simulink model "HybridEngModel"  (R2013a)
settings: Solver=ode15s  StartTime=0  StopTime=100  FixedStep=1e-3  RelTol=1e-5  AbsTol=1e-5
values from neighbouring files (symbols this model uses):
  B = [B1;B2]    [GensetRespOptimiztion.m]    (also in GensetRespOptimiztionTorstein.m; Init8RTFLEX68D.m = 0.68; init_MVM.m = 0.127)
  beta = 0.75    [Init8RTFLEX68D.m]
  cAStartRef = 104.8    [Init8RTFLEX68D.m]
  dCALiftDown = cAVVDownRef(end) - cAVVDownRef(1)    [Init8RTFLEX68D.m]
  dCALiftTopRef = 63.5    [Init8RTFLEX68D.m]
  dCALiftUp = cAVVUpRef(end) - cAVVUpRef(1)    [Init8RTFLEX68D.m]
  Dp = 0.383    [Init8RTFLEX68D.m]
  Ds = 0.079    [Init8RTFLEX68D.m]
  Dv = 0.425    [Init8RTFLEX68D.m]
  liftMax = 0.17    [Init8RTFLEX68D.m]
  nStroke = 2    [Init8RTFLEX68D.m]
  w = 0.021    [Init8RTFLEX68D.m]
  wNL0 = 1./(1-Droop*.5)    [initHybrid.m]    (also in initMV.m; init_ele.m = 1.0101010101)
undefined symbols (not defined in the file or in its folder): cAVVDownRef, cAVVUpRef, generators, liftDownRef, liftUpRef
undefined symbols (not defined in the file): aCrank, cAlpha, cCylHT, E0A, ECyl0, fs, hn, lambdaCrank, m0A, mb0A, mbCyl0, mCp, mCyl0, mqfCycMax, nCyl, nPort, phi0, phi0A, r, stroke, V0A, vCyl0, wiebePara, X, Y
libraries: EngineSystemSubmodel x15, simulink x1, gensetMV x1
settings Model: Creator=yum  LastModifiedBy=yum
settings DataIOCC: SaveFormat=StructureWithTime  InspectSignalLogs=on  ReturnWorkspaceOutputs=on
settings DebuggingCC: SolverPrmCheckMsg=none

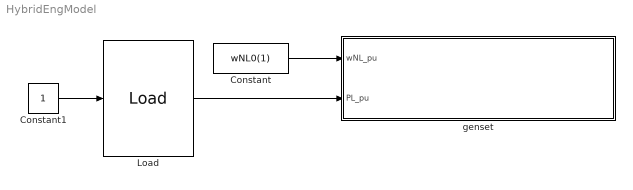
== system HybridEngModel ==
  Constant : Constant  Value=wNL0(1)
  Constant1 : Constant
  Load : EngineSystemSubmodel/Load  Load_index=Load_index  Load_amp=Load_amp  Load_bias=Load_bias  Start_time=Start_time  T_load=T_load
  genset : Subsystem  mask{genset=generators(1)}
      mask prompts: genset "Generator parameters"
  wires:
  Load/1 -> genset/2(PL_pu)
  Constant/1 -> genset/1(wNL_pu)
  Constant1/1 -> Load/1

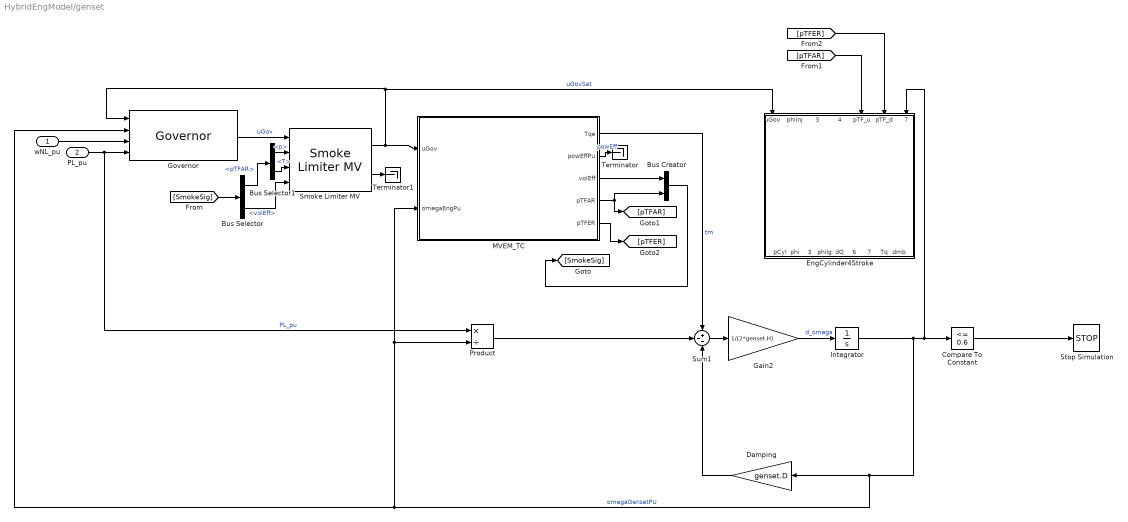
== system HybridEngModel/genset ==
  wNL_pu : Inport
  PL_pu : Inport  Port=2
  Bus Creator : BusCreator  Inputs=2
  Bus Selector : BusSelector  OutputSignals=pTFAR,volEff
  Bus Selector1 : BusSelector  OutputSignals=p,T
  Compare To Constant : simulink/Logic and Bit Operations/Compare To Constant  relop=<=  const=0.6  OutDataTypeStr=boolean
  Damping : Gain  Gain=genset.D
  EngCylinder4Stroke : Subsystem  mask{fs=fs, nStroke=nStroke, hn=hn, nCyl=nCyl, iCyl=2, B=B, stroke=stroke, lambdaCrank=lambdaCrank, aCrank=aCrank, X=X, Y=Y, r=r, nPort=nPort, liftMax=liftMax, Dv=Dv, beta=beta, w=w, Dp=Dp, Ds=Ds, cAVVUpRef=cAVVUpRef, cAVVDownRef=cAVVDownRef, liftUpRef=liftUpRef, liftDownRef=liftDownRef, cAStartRef=cAStartRef, dCALiftUp=dCALiftUp, dCALiftDown=dCALiftDown, dCALiftTopRef=dCALiftTopRef, mCp=mCp, cCylHT=cCylHT, cAlpha=cAlpha, mqfCycMax=mqfCycMax, wiebePara=wiebePara, phi0=phi0, m0=mCyl0, E0=ECyl0, mb0=mbCyl0, V0=vCyl0, phi0A=phi0A, m0A=m0A, E0A=E0A, mb0A=mb0A, V0A=V0A}
      mask prompts: fs "Stoichiometric fuel-air ratio"; nStroke "Number of stroke"; hn "Lower heating value of the fuel [J/kg]"; nCyl "Number of cylinders"; iCyl "Cylinder number"; B "Bore of the cylinder [m]"; stroke "Stroke [m]"; lambdaCrank "Ratio of length of crank rod to connecting rod"; aCrank "Length of crank rod [m]"; X "Width of inport opening [m]"; Y "Height of inport opening [m]"; r "Raidus of fillet of the opening"; nPort "Number of ports [pcs]"; liftMax "Maximum valve lift [m]"; Dv "Valve head diameter [m]"; beta "Seat angle [rad]"; w "Valve seat width [m]"; Dp "Inner seat diameter [m]"; Ds "Stem diameter [m]"; cAVVUpRef "Crank angle array for opening [deg]"; cAVVDownRef "Crank angle array for closing [deg]"; liftUpRef "Normalized lift array for opening (0~1)"; liftDownRef "Normalized lift array for closing (0~1)"; cAStartRef "Nominal crank angle at start of valve lif [deg]"; dCALiftUp "Nominal duration of crank angle for valve opening [deg]"; dCALiftDown "Nominal duration of crank angle for valve closing [deg]"; dCALiftTopRef "Nominal duration of crank angle for valve open [deg]"; mCp "Heat capacity of the cylinder [J/K]"; cCylHT "Polynomial coefficient for heat rejection model from the cylinder (4 x 1)"; cAlpha "Fitting coefficient for convective heat transfer coefficient"; mqfCycMax "Maximum fuel mass injected per cycle [kg]"; wiebePara "3-Wiebe Parameters (9x1)"; phi0 "Initial crank angle [deg]"; m0 "Initial mass [kg]"; E0 "Initial internal energy [J]"; mb0 "Initial burned fuel mass [kg]"; V0 "Initial volume [m3]"; phi0A "Initial crank angle array [deg]"; m0A "Initial mass array [kg]"; E0A "Initial internal energy array [J]"; mb0A "Initial burned fuel mass array [kg]"; V0A "Initial volume array [m3]"
      mask init:
      | CylNo = uint8(iCyl);
      | if CylNo > 0 
      |     phi0 = phi0A(CylNo);
      |     m0 = m0A(CylNo);
      |     E0 = E0A(CylNo);
      |     mb0 = mb0A(CylNo);
      |     V0 = V0A(CylNo);
      | else
      |     phi0 = phi0A(1);
      |     m0 = m0A(1);
      |     E0 = E0A(1);
      |     mb0 = mb0A(1);
      |     V0 = V0A(1);
      | end;
      mask TypeOptions fs: ThdynCV_VarVol1/fs | IntakePort1/fs | ExhValve/fs
      mask TypeOptions nStroke: IntakePort1/nStroke
      mask TypeOptions hn: ROHR1/hn
      mask TypeOptions nCyl: EngCylHeatTransfer/nCyl
      mask TypeOptions B: CrankMechKinematic/B | EngCylHeatTransfer/B
      mask TypeOptions stroke: CrankMechKinematic/stroke | EngCylHeatTransfer/stroke | IntakePort1/stroke
      mask TypeOptions lambdaCrank: IntakePort1/lambdaCrank | CrankMechKinematic/lambdaCrank
      mask TypeOptions aCrank: IntakePort1/aCrank
      mask TypeOptions X: IntakePort1/X
      mask TypeOptions Y: IntakePort1/Y
      mask TypeOptions r: IntakePort1/r
      mask TypeOptions nPort: IntakePort1/nPort
      mask TypeOptions liftMax: ExhValve/liftMax
      mask TypeOptions Dv: ExhValve/Dv
      mask TypeOptions beta: ExhValve/beta
      mask TypeOptions w: ExhValve/w
      mask TypeOptions Dp: ExhValve/Dp
      mask TypeOptions Ds: ExhValve/Ds
      mask TypeOptions cAVVUpRef: ExhValve/cAVVUpRef
      mask TypeOptions cAVVDownRef: ExhValve/cAVVDownRef
      mask TypeOptions liftUpRef: ExhValve/liftUpRef
      mask TypeOptions liftDownRef: ExhValve/liftDownRef
      mask TypeOptions cAStartRef: ExhValve/cAStartRef
      mask TypeOptions dCALiftUp: ExhValve/dCALiftUp
      mask TypeOptions dCALiftDown: ExhValve/dCALiftDown
      mask TypeOptions dCALiftTopRef: ExhValve/dCALiftTopRef
      mask TypeOptions mCp: EngCylHeatTransfer/mCp
      mask TypeOptions cCylHT: EngCylHeatTransfer/cCylHT
      mask TypeOptions cAlpha: EngCylHeatTransfer/cAlpha
      mask TypeOptions mqfCycMax: ROHR1/mqfCycMax
      mask TypeOptions wiebePara: ROHR1/wiebePara
      mask TypeOptions phi0: CrankMechKinematic/phi0
      mask TypeOptions m0: ThdynCV_VarVol1/m0
      mask TypeOptions E0: ThdynCV_VarVol1/E0
      mask TypeOptions mb0: ThdynCV_VarVol1/mb0
      mask TypeOptions V0: ThdynCV_VarVol1/V0
  Gain2 : Gain  Gain=1/(2*genset.H)
  Governor : gensetMV/GensetAC_MVM/Genset/Governor
  Integrator : Integrator  InitialCondition=generators(1).omega0
  MVEM_TC : Subsystem  mask{genset=genset}
      mask prompts: genset "Genset parameters"
  Product : Product  Inputs=*/
  Smoke Limiter MV : EngineSystemSubmodel/Smoke Limiter MV  fs=genset.eng.fs  Vd=genset.eng.vD  F_max=genset.eng.fMax  m_f_cyc_max=genset.eng.mFCycMax
  Stop Simulation : Stop
  Sum1 : Sum  Inputs=+--
  Terminator : Terminator
  Terminator1 : Terminator
  wires:
  Sum1/1 -> Gain2/1
  Gain2/1 -> Integrator/1  "d_omega"
  MVEM_TC/4(pTFAR) -> Bus Creator/2, [pTFAR]
  Governor/1 -> Smoke Limiter MV/1  "uGov"
  Integrator/1 -> EngCylinder4Stroke/7(omega), Compare To Constant/1, Governor/2, MVEM_TC/2(omegaEngPu), Product/2, Damping/1  "omegaGensetPU"
  MVEM_TC/2(powEffPu) -> Terminator/1  "powEff"
  Smoke Limiter MV/2 -> Terminator1/1
  wNL_pu/1 -> Governor/3
  MVEM_TC/1(Tqe) -> Sum1/1  "tm"
  Damping/1 -> Sum1/3
  Bus Creator/1 -> [SmokeSig]
  Product/1 -> Sum1/2
  PL_pu/1 -> Product/1, Governor/4  "PL_pu"
  Smoke Limiter MV/1 -> MVEM_TC/1(uGov), EngCylinder4Stroke/1(uGov), Governor/1  "uGovSat"
  [SmokeSig] -> Bus Selector/1
  Bus Selector/2 -> Smoke Limiter MV/4  "<volEff>"
  MVEM_TC/3(volEff) -> Bus Creator/1
  Compare To Constant/1 -> Stop Simulation/1
  Bus Selector/1 -> Bus Selector1/1  "<pTFAR>"
  Bus Selector1/1 -> Smoke Limiter MV/2  "<p>"
  Bus Selector1/2 -> Smoke Limiter MV/3  "<T>"
  MVEM_TC/5(pTFER) -> [pTFER]
  [pTFAR] -> EngCylinder4Stroke/5(pTF_u)
  [pTFER] -> EngCylinder4Stroke/6(pTF_d)

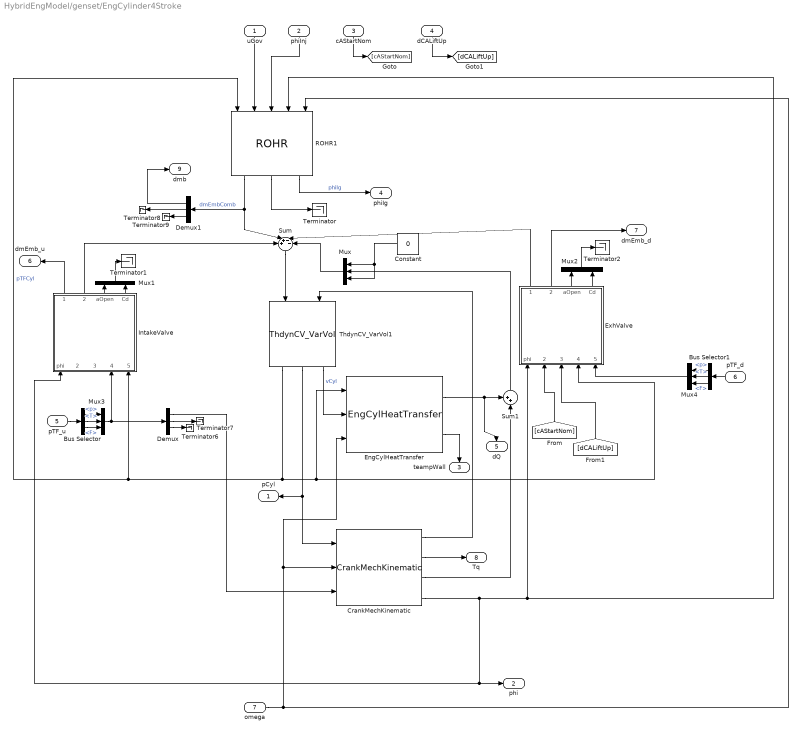
== system HybridEngModel/genset/EngCylinder4Stroke ==
  uGov : Inport
  phiInj : Inport  Port=2
  cAStartNom : Inport  Port=3
  dCALiftUp : Inport  Port=4
  pTF_u : Inport  Port=5
  pTF_d : Inport  Port=6
  omega : Inport  Port=7
  Bus Selector : BusSelector  OutputSignals=p,T,F
  Bus Selector1 : BusSelector  OutputSignals=p,T,F
  Constant : Constant  Value=0
  CrankMechKinematic : EngineSystemSubmodel/CrankMechKinematic  phi0=phi0  B=B  stroke=stroke  lambdaCrank=lambdaCrank
  Demux : Demux  Outputs=3
  Demux1 : Demux  Outputs=3
  EngCylHeatTransfer : EngineSystemSubmodel/EngCylHeatTransfer  stroke=stroke  B=B  cAlpha=cAlpha  mCp=mCp  cCylHT=cCylHT  nCyl=nCyl  tempWall0=600
  ExhValve : Subsystem  mask{fs=fs, cAVVUpRef=cAVVUpRef, cAVVDownRef=cAVVDownRef, liftUpRef=liftUpRef, liftDownRef=liftDownRef, cAStartRef=cAStartRef, dCALiftUp=dCALiftUp, dCALiftDown=dCALiftDown, dCALiftTopRef=dCALiftTopRef, liftMax=liftMax, Dv=Dv, beta=beta, w=w, Dp=Dp, Ds=Ds}
      mask prompts: fs "Stoichiometric fuel-air equivalent ratio"; cAVVUpRef "Crank angle array for opening [deg]"; cAVVDownRef "Crank angle array for closing [deg]"; liftUpRef "Normalized lift array for opening (0~1)"; liftDownRef "Normalized lift array for closing (0~1)"; cAStartRef "Nominal crank angle at start of valve lif [deg]"; dCALiftUp "Nominal duration of crank angle for valve opening [deg]"; dCALiftDown "Nominal duration of crank angle for valve closing [deg]"; dCALiftTopRef "Nominal duration of crank angle for valve open [deg]"; liftMax "Maximum valve lift [m]"; Dv "Valve head diameter [m]"; beta "Seat angle [rad]"; w "Valve seat width [m]"; Dp "Inner seat diameter [m]"; Ds "Stem diameter [m]"
      mask TypeOptions fs: IdealNozzle/fs
      mask TypeOptions cAVVUpRef: S-Function/cAVVUpRef
      mask TypeOptions cAVVDownRef: S-Function/cAVVDownRef
      mask TypeOptions liftUpRef: S-Function/liftUpRef
      mask TypeOptions liftDownRef: S-Function/liftDownRef
      mask TypeOptions cAStartRef: S-Function/cAStartRef
      mask TypeOptions dCALiftUp: S-Function/dCALiftUp
      mask TypeOptions dCALiftDown: S-Function/dCALiftDown
      mask TypeOptions dCALiftTopRef: S-Function/dCALiftTopRef
      mask TypeOptions liftMax: S-Function/liftMax
      mask TypeOptions Dv: S-Function1/Dv
      mask TypeOptions beta: S-Function1/beta
      mask TypeOptions w: S-Function1/w
      mask TypeOptions Dp: S-Function1/Dp
      mask TypeOptions Ds: S-Function1/Ds
  IntakeValve : Subsystem  mask{fs=0, cAVVUpRef=0, cAVVDownRef=0, liftUpRef=0, liftDownRef=0, cAStartRef=0, dCALiftUp=0, dCALiftDown=0, dCALiftTopRef=0, liftMax=0, Dv=0, beta=0, w=0, Dp=0, Ds=0}
      mask prompts: fs "Stoichiometric fuel-air equivalent ratio"; cAVVUpRef "Crank angle array for opening [deg]"; cAVVDownRef "Crank angle array for closing [deg]"; liftUpRef "Normalized lift array for opening (0~1)"; liftDownRef "Normalized lift array for closing (0~1)"; cAStartRef "Nominal crank angle at start of valve lif [deg]"; dCALiftUp "Nominal duration of crank angle for valve opening [deg]"; dCALiftDown "Nominal duration of crank angle for valve closing [deg]"; dCALiftTopRef "Nominal duration of crank angle for valve open [deg]"; liftMax "Maximum valve lift [m]"; Dv "Valve head diameter [m]"; beta "Seat angle [rad]"; w "Valve seat width [m]"; Dp "Inner seat diameter [m]"; Ds "Stem diameter [m]"
      mask TypeOptions fs: IdealNozzle/fs
      mask TypeOptions cAVVUpRef: S-Function/cAVVUpRef
      mask TypeOptions cAVVDownRef: S-Function/cAVVDownRef
      mask TypeOptions liftUpRef: S-Function/liftUpRef
      mask TypeOptions liftDownRef: S-Function/liftDownRef
      mask TypeOptions cAStartRef: S-Function/cAStartRef
      mask TypeOptions dCALiftUp: S-Function/dCALiftUp
      mask TypeOptions dCALiftDown: S-Function/dCALiftDown
      mask TypeOptions dCALiftTopRef: S-Function/dCALiftTopRef
      mask TypeOptions liftMax: S-Function/liftMax
      mask TypeOptions Dv: S-Function1/Dv
      mask TypeOptions beta: S-Function1/beta
      mask TypeOptions w: S-Function1/w
      mask TypeOptions Dp: S-Function1/Dp
      mask TypeOptions Ds: S-Function1/Ds
  Mux : Mux  Inputs=3
  Mux1 : Mux  Inputs=2
  Mux2 : Mux  Inputs=2
  Mux3 : Mux  Inputs=3
  Mux4 : Mux  Inputs=3
  ROHR1 : EngineSystemSubmodel/ROHR  mqfCycMax=mqfCycMax  wiebePara=wiebePara  hn=hn
  Sum : Sum  Inputs=++--
  Sum1 : Sum  Inputs=++|
  Terminator{,1..2,6..9} (7 alike) : Terminator
  ThdynCV_VarVol1 : EngineSystemSubmodel/ThdynCV_VarVol  fs=fs  m0=m0  E0=E0  mb0=mb0  V0=V0
  pCyl : Outport
  phi : Outport  Port=2
  teampWall : Outport  Port=3
  phiIg : Outport  Port=4
  dQ : Outport  Port=5
  dmEmb_u : Outport  Port=6
  dmEmb_d : Outport  Port=7
  Tq : Outport  Port=8
  dmb : Outport  Port=9
  wires:
  Demux1/3 -> Terminator9/1
  Demux1/2 -> Terminator8/1
  Demux1/1 -> dmb/1
  ROHR1/1 -> Demux1/1, Sum/2  "dmEmbComb"
  IntakeValve/2(dmEmb_d) -> Sum/1
  ExhValve/1(dmEmb_u) -> Sum/3
  Sum/1 -> ThdynCV_VarVol1/1
  ThdynCV_VarVol1/1 -> EngCylHeatTransfer/1, ExhValve/4(pTF_u), ROHR1/1, IntakeValve/5(pTF_d)  "pTFCyl"
  ThdynCV_VarVol1/2 -> pCyl/1, CrankMechKinematic/1
  CrankMechKinematic/4 -> ROHR1/4, ExhValve/1(phi), IntakeValve/1(phi), phi/1
  CrankMechKinematic/1 -> ThdynCV_VarVol1/2
  uGov/1 -> ROHR1/2
  CrankMechKinematic/3 -> Sum1/2
  Demux/1 -> CrankMechKinematic/3
  CrankMechKinematic/2 -> Tq/1
  phiInj/1 -> ROHR1/3
  omega/1 -> EngCylHeatTransfer/3, CrankMechKinematic/2, ROHR1/5
  ROHR1/2 -> Terminator/1
  IntakeValve/1(dmEmb_u) -> dmEmb_u/1
  ThdynCV_VarVol1/3 -> EngCylHeatTransfer/2  "vCyl"
  EngCylHeatTransfer/1 -> Sum1/1, dQ/1
  Sum1/1 -> Mux/2
  Mux/1 -> Sum/4
  Constant/1 -> Mux/3, Mux/1
  Demux/2 -> Terminator6/1
  Demux/3 -> Terminator7/1
  EngCylHeatTransfer/2 -> teampWall/1
  ROHR1/3 -> phiIg/1  "phiIg"
  Mux1/1 -> Terminator1/1
  ExhValve/3(aOpen) -> Mux2/1
  ExhValve/4(Cd) -> Mux2/2
  Mux2/1 -> Terminator2/1
  ExhValve/2(dmEmb_d) -> dmEmb_d/1
  cAStartNom/1 -> [cAStartNom]
  dCALiftUp/1 -> [dCALiftUp]
  [cAStartNom] -> ExhValve/2(cAStartNom)
  [dCALiftUp] -> ExhValve/3(dCALiftUp)
  IntakeValve/3(aOpen) -> Mux1/1
  IntakeValve/4(Cd) -> Mux1/2
  pTF_u/1 -> Bus Selector/1
  Bus Selector/3 -> Mux3/3  "<F>"
  Bus Selector/2 -> Mux3/2  "<T>"
  Bus Selector/1 -> Mux3/1  "<p>"
  Mux3/1 -> Demux/1, IntakeValve/4(pTF_u)
  pTF_d/1 -> Bus Selector1/1
  Bus Selector1/3 -> Mux4/3  "<F>"
  Bus Selector1/2 -> Mux4/2  "<T>"
  Bus Selector1/1 -> Mux4/1  "<p>"
  Mux4/1 -> ExhValve/5(pTF_d)

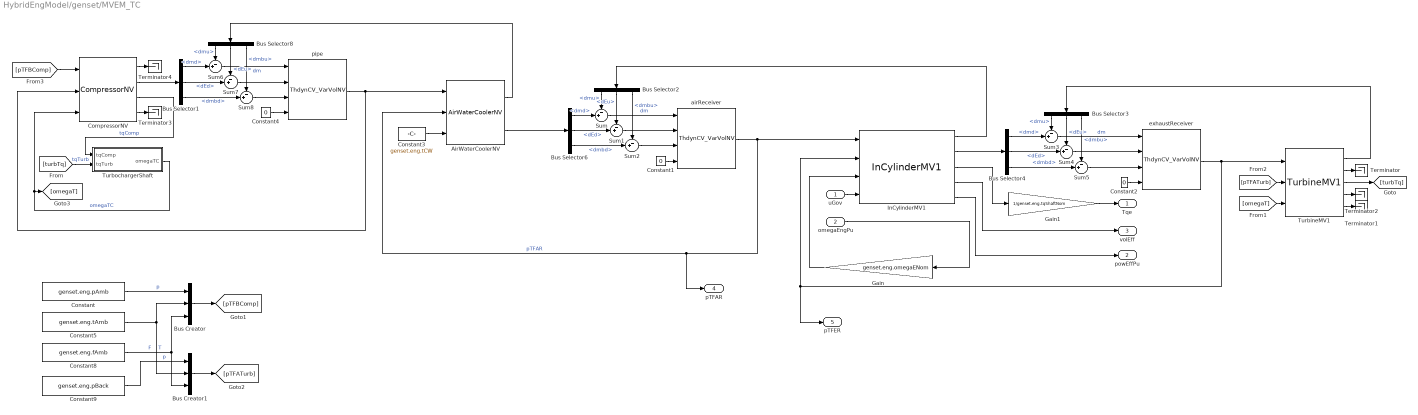
== system HybridEngModel/genset/MVEM_TC ==
  uGov : Inport
  omegaEngPu : Inport  Port=2
  AirWaterCoolerNV : EngineSystemSubmodel/AirWaterCoolerNV  fs=genset.eng.fs  Cd=genset.eng.cdCool  A_air_path=genset.eng.aAirPath  dm_cw=genset.eng.dmCW  coeff_T_cw_K=genset.eng.coeffKTCW  Cp_cw=genset.eng.cpCW  D_cw_pipe=genset.eng.dPipeCW
  Bus Creator : BusCreator  Inputs=3
  Bus Creator1 : BusCreator  Inputs=3
  Bus Selector1 : BusSelector  OutputSignals=dmd,dEd,dmbd
  Bus Selector2 : BusSelector  OutputSignals=dmu,dEu,dmbu
  Bus Selector3 : BusSelector  OutputSignals=dmu,dEu,dmbu
  Bus Selector4 : BusSelector  OutputSignals=dmd,dEd,dmbd
  Bus Selector6 : BusSelector  OutputSignals=dmd,dEd,dmbd
  Bus Selector8 : BusSelector  OutputSignals=dmu,dEu,dmbu
  CompressorNV : EngineSystemSubmodel/CompressorNV  fs=genset.eng.fs  comp_flow_map=genset.eng.compFlowMap  comp_eff_map=genset.eng.compEffMap  pr_rep=genset.eng.prRep  n288_rep=genset.eng.n288Rep  npr=genset.eng.npr  nsp=genset.eng.nsp
  Constant : Constant  Value=genset.eng.pAmb
  Constant1 : Constant  Value=0
  Constant2 : Constant  Value=0
  Constant3 : Constant  Value=genset.eng.tCW
  Constant4 : Constant  Value=0
  Constant5 : Constant  Value=genset.eng.tAmb
  Constant8 : Constant  Value=genset.eng.fAmb
  Constant9 : Constant  Value=genset.eng.pBack
  Gain : Gain  Gain=genset.eng.omegaENom
  Gain1 : Gain  Gain=1/genset.eng.tqShaftNom
  InCylinderMV1 : EngineSystemSubmodel/InCylinderMV1  fs=genset.eng.fs  Vd=genset.eng.vD  LHV=genset.eng.LHV  Pe_nom=genset.eng.powNom  SFC=genset.eng.SFC  vol_eff_coeff1=genset.eng.volEff1  vol_eff_coeff2=genset.eng.volEff2  T_pe=genset.eng.tPe  nstroke=genset.eng.nStroke  m_f_cyc_max=genset.eng.mFCycMax  C1=genset.eng.C1  p_a_inf=genset.eng.pAInf  Pe0=genset.eng.powL0*genset.eng.powNom
  Sum{,1..8} (9 alike) : Sum  Inputs=-+|
  Terminator{,1..4} (5 alike) : Terminator
  TurbineMV1 : EngineSystemSubmodel/TurbineMV1  fs=genset.eng.fs  flow_coeff_turb=genset.eng.flowCoeffTurb  D_turb_wheel=genset.eng.dTurbWheel  Uc_opt=genset.eng.ucOpt  eta_turb_max=genset.eng.effTurbMax
  TurbochargerShaft : Subsystem
  airReceiver : EngineSystemSubmodel/ThdynCV_VarVolNV  fs=genset.eng.fs  m0=genset.eng.m0AR  E0=genset.eng.E0AR  mb0=genset.eng.mb0AR  V0=genset.eng.vAR
  exhaustReceiver : EngineSystemSubmodel/ThdynCV_VarVolNV  fs=genset.eng.fs  m0=genset.eng.m0ER  E0=genset.eng.E0ER  mb0=genset.eng.mb0ER  V0=genset.eng.vER
  pipe : EngineSystemSubmodel/ThdynCV_VarVolNV  fs=genset.eng.fs  m0=genset.eng.m0PipeAComp  E0=genset.eng.e0PipeAComp  mb0=genset.eng.mb0PipeAComp  V0=genset.eng.vPipeAComp
  Tqe : Outport
  powEffPu : Outport  Port=2
  volEff : Outport  Port=3
  pTFAR : Outport  Port=4
  pTFER : Outport  Port=5
  wires:
  TurbochargerShaft/1(omegaTC) -> [omegaT], CompressorNV/3  "omegaTC"
  [turbTq] -> TurbochargerShaft/2(tqTurb)  "tqTurb"
  CompressorNV/3 -> TurbochargerShaft/1(tqComp)  "tqComp"
  InCylinderMV1/3 -> Gain1/1
  CompressorNV/1 -> Terminator4/1
  CompressorNV/4 -> Terminator3/1
  Gain1/1 -> Tqe/1
  uGov/1 -> InCylinderMV1/4
  InCylinderMV1/4 -> volEff/1
  Constant3/1 -> AirWaterCoolerNV/3
  CompressorNV/2 -> Bus Selector1/1
  Bus Selector4/1 -> Sum3/2  "<dmd>"
  Constant1/1 -> airReceiver/4
  Bus Selector4/3 -> Sum5/2  "<dmbd>"
  Bus Selector6/3 -> Sum2/2  "<dmbd>"
  InCylinderMV1/2 -> Bus Selector4/1
  Sum4/1 -> exhaustReceiver/2
  Bus Selector4/2 -> Sum4/2  "<dEd>"
  Sum2/1 -> airReceiver/3
  Sum1/1 -> airReceiver/2
  Sum5/1 -> exhaustReceiver/3
  Constant2/1 -> exhaustReceiver/4
  Sum3/1 -> exhaustReceiver/1  "dm"
  Bus Selector6/2 -> Sum1/2  "<dEd>"
  Bus Selector6/1 -> Sum/2  "<dmd>"
  AirWaterCoolerNV/1 -> Bus Selector8/1
  Bus Selector8/3 -> Sum8/1  "<dmbu>"
  pipe/1 -> AirWaterCoolerNV/1, CompressorNV/2
  Sum8/1 -> pipe/3
  Gain/1 -> InCylinderMV1/3
  Bus Selector8/1 -> Sum6/1  "<dmu>"
  Sum7/1 -> pipe/2
  Bus Selector8/2 -> Sum7/1  "<dEu>"
  AirWaterCoolerNV/2 -> Bus Selector6/1
  Sum6/1 -> pipe/1  "dm"
  InCylinderMV1/5 -> powEffPu/1
  TurbineMV1/1 -> Bus Selector3/1
  [omegaT] -> TurbineMV1/3
  Bus Selector3/1 -> Sum3/1  "<dmu>"
  Bus Creator/1 -> [pTFBComp]
  Bus Selector1/1 -> Sum6/2  "<dmd>"
  Bus Selector1/3 -> Sum8/2  "<dmbd>"
  Bus Selector1/2 -> Sum7/2  "<dEd>"
  Constant4/1 -> pipe/4
  airReceiver/1 -> pTFAR/1, AirWaterCoolerNV/2, InCylinderMV1/1  "pTFAR"
  omegaEngPu/1 -> Gain/1
  exhaustReceiver/1 -> pTFER/1, InCylinderMV1/2, TurbineMV1/1
  Bus Selector2/3 -> Sum2/1  "<dmbu>"
  Bus Selector2/2 -> Sum1/1  "<dEu>"
  Sum/1 -> airReceiver/1  "dm"
  Bus Selector2/1 -> Sum/1  "<dmu>"
  InCylinderMV1/1 -> Bus Selector2/1
  Bus Selector3/3 -> Sum5/1  "<dmbu>"
  TurbineMV1/3 -> [turbTq]
  [pTFATurb] -> TurbineMV1/2
  [pTFBComp] -> CompressorNV/1
  Bus Selector3/2 -> Sum4/1  "<dEu>"
  Constant9/1 -> Bus Creator1/1  "p"
  Bus Creator1/1 -> [pTFATurb]
  Constant/1 -> Bus Creator/1  "p"
  Constant8/1 -> Bus Creator/3, Bus Creator1/3  "F"
  Constant5/1 -> Bus Creator/2, Bus Creator1/2  "T"
  TurbineMV1/5 -> Terminator1/1
  TurbineMV1/4 -> Terminator2/1
  TurbineMV1/2 -> Terminator/1

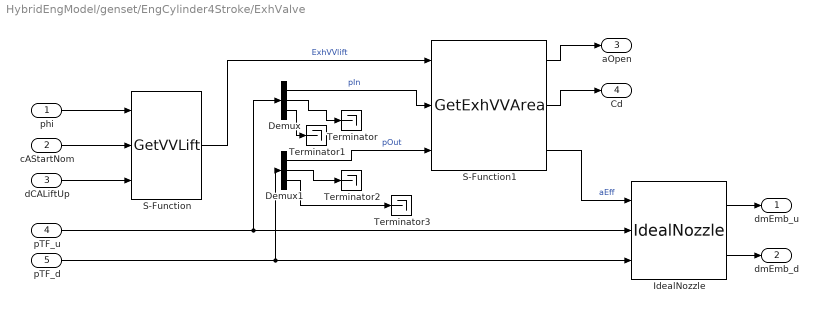
== system HybridEngModel/genset/EngCylinder4Stroke/ExhValve ==
  phi : Inport
  cAStartNom : Inport  Port=2
  dCALiftUp : Inport  Port=3
  pTF_u : Inport  Port=4
  pTF_d : Inport  Port=5
  Demux : Demux  Outputs=3
  Demux1 : Demux  Outputs=3
  IdealNozzle : EngineSystemSubmodel/IdealNozzle  fs=fs
  S-Function : S-Function  FunctionName=GetVVLift  Parameters=nStroke,liftMax,cAStartRef,dCALiftUp,dCALiftDown,dCALiftTopRef,cAVVUpRef,cAVVDownRef,liftUpRef,liftDownRef  EnableBusSupport=off  mask{nStroke=nStroke, liftMax=liftMax, cAStartRef=cAStartRef, dCALiftUp=dCALiftUp, dCALiftDown=dCALiftDown, dCALiftTopRef=dCALiftTopRef, cAVVUpRef=cAVVUpRef, cAVVDownRef=cAVVDownRef, liftUpRef=liftUpRef, liftDownRef=liftDownRef}
      mask prompts: nStroke "Number of stroke"; liftMax "Maximum valve lift [m]"; cAStartRef "Crank angle at the beginning of valve lift [deg]"; dCALiftUp "Duration for valve lifting [deg]"; dCALiftDown "Duration for valve closing [deg]"; dCALiftTopRef "Duration for valve fully opened [deg]"; cAVVUpRef "Crank angle array reference for valve opening [deg]"; cAVVDownRef "Crank angle array reference for valve closing [deg]"; liftUpRef "Normalized lift reference for valve opening (0~1)"; liftDownRef "Normalized lift reference for valve closing (0~1)"
  S-Function1 : S-Function  FunctionName=GetExhVVArea  Parameters=Dv,beta,w,Dp,Ds,coeffCdCorrP,coeffCdCorrQ,coeffCdCorrPR  EnableBusSupport=off  mask{Dv=Dv, beta=beta, w=w, Dp=Dp, Ds=Ds, coeffCdCorrP=[0.5329;-0.2047;0.04292], coeffCdCorrQ=[0.5359;-0.2962;0.06275], coeffCdCorrPR=[-0.006345;0.09503;0.8117]}
      mask prompts: Dv "Valve head diameter"; beta "Seat angle"; w "Valve seat width"; Dp "Inner seat diameter"; Ds "Stem diameter"; coeffCdCorrP "Produt coefficient for discharge coefficient for lift ratio"; coeffCdCorrQ "Quotient coefficient for discharge coefficient for lift ratio"; coeffCdCorrPR "Coefficient for discharge coefficient for pressure ratio"
  Terminator{,1..3} (4 alike) : Terminator
  dmEmb_u : Outport
  dmEmb_d : Outport  Port=2
  aOpen : Outport  Port=3
  Cd : Outport  Port=4
  wires:
  S-Function/1 -> S-Function1/1  "ExhVVlift"
  pTF_d/1 -> Demux1/1, IdealNozzle/3
  pTF_u/1 -> Demux/1, IdealNozzle/2
  IdealNozzle/2 -> dmEmb_d/1
  IdealNozzle/1 -> dmEmb_u/1
  phi/1 -> S-Function/1
  cAStartNom/1 -> S-Function/2
  dCALiftUp/1 -> S-Function/3
  S-Function1/3 -> IdealNozzle/1  "aEff"
  S-Function1/1 -> aOpen/1
  S-Function1/2 -> Cd/1
  Demux/1 -> S-Function1/2  "pIn"
  Demux1/1 -> S-Function1/3  "pOut"
  Demux/2 -> Terminator/1
  Demux/3 -> Terminator1/1
  Demux1/2 -> Terminator2/1
  Demux1/3 -> Terminator3/1

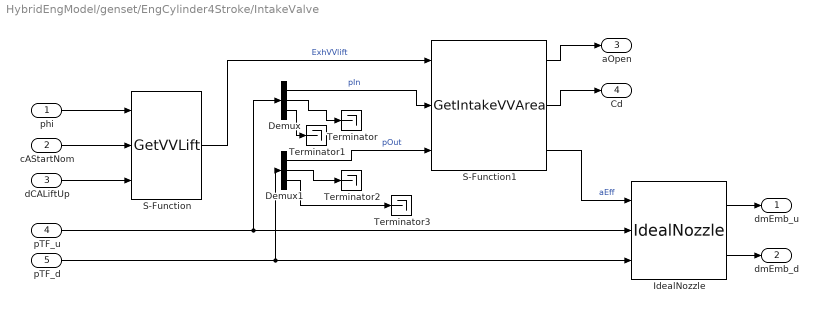
== system HybridEngModel/genset/EngCylinder4Stroke/IntakeValve ==
  phi : Inport
  cAStartNom : Inport  Port=2
  dCALiftUp : Inport  Port=3
  pTF_u : Inport  Port=4
  pTF_d : Inport  Port=5
  Demux : Demux  Outputs=3
  Demux1 : Demux  Outputs=3
  IdealNozzle : EngineSystemSubmodel/IdealNozzle  fs=fs
  S-Function : S-Function  FunctionName=GetVVLift  Parameters=nStroke,liftMax,cAStartRef,dCALiftUp,dCALiftDown,dCALiftTopRef,cAVVUpRef,cAVVDownRef,liftUpRef,liftDownRef  EnableBusSupport=off  mask{nStroke=0, liftMax=liftMax, cAStartRef=cAStartRef, dCALiftUp=dCALiftUp, dCALiftDown=dCALiftDown, dCALiftTopRef=dCALiftTopRef, cAVVUpRef=cAVVUpRef, cAVVDownRef=cAVVDownRef, liftUpRef=liftUpRef, liftDownRef=liftDownRef}
      mask prompts: nStroke "Number of stroke"; liftMax "Maximum valve lift [m]"; cAStartRef "Crank angle at the beginning of valve lift [deg]"; dCALiftUp "Duration for valve lifting [deg]"; dCALiftDown "Duration for valve closing [deg]"; dCALiftTopRef "Duration for valve fully opened [deg]"; cAVVUpRef "Crank angle array reference for valve opening [deg]"; cAVVDownRef "Crank angle array reference for valve closing [deg]"; liftUpRef "Normalized lift reference for valve opening (0~1)"; liftDownRef "Normalized lift reference for valve closing (0~1)"
  S-Function1 : S-Function  FunctionName=GetIntakeVVArea  Parameters=Dv,beta,w,Dp,Ds  EnableBusSupport=off  mask{Dv=Dv, beta=beta, w=w, Dp=Dp, Ds=Ds}
      mask prompts: Dv "Valve head diameter"; beta "Seat angle"; w "Valve seat width"; Dp "Inner seat diameter"; Ds "Stem diameter"
  Terminator{,1..3} (4 alike) : Terminator
  dmEmb_u : Outport
  dmEmb_d : Outport  Port=2
  aOpen : Outport  Port=3
  Cd : Outport  Port=4
  wires:
  S-Function/1 -> S-Function1/1  "ExhVVlift"
  pTF_d/1 -> Demux1/1, IdealNozzle/3
  pTF_u/1 -> Demux/1, IdealNozzle/2
  IdealNozzle/2 -> dmEmb_d/1
  IdealNozzle/1 -> dmEmb_u/1
  phi/1 -> S-Function/1
  cAStartNom/1 -> S-Function/2
  dCALiftUp/1 -> S-Function/3
  S-Function1/3 -> IdealNozzle/1  "aEff"
  S-Function1/1 -> aOpen/1
  S-Function1/2 -> Cd/1
  Demux/1 -> S-Function1/2  "pIn"
  Demux1/1 -> S-Function1/3  "pOut"
  Demux/2 -> Terminator/1
  Demux/3 -> Terminator1/1
  Demux1/2 -> Terminator2/1
  Demux1/3 -> Terminator3/1

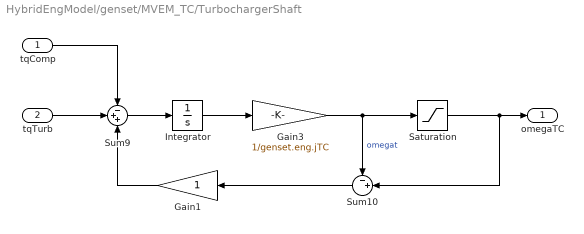
== system HybridEngModel/genset/MVEM_TC/TurbochargerShaft ==
  tqComp : Inport
  tqTurb : Inport  Port=2
  Gain1 : Gain
  Gain3 : Gain  Gain=1/genset.eng.jTC
  Integrator : Integrator  InitialCondition=genset.eng.omegaT0*genset.eng.jTC
  Saturation : Saturate  UpperLimit=genset.eng.RPMtMax*pi/30*1.1;  LowerLimit=genset.eng.RPMtMax*pi/30*0.24;
  Sum10 : Sum  Inputs=-+|
  Sum9 : Sum  Inputs=-++
  omegaTC : Outport
  wires:
  Gain1/1 -> Sum9/3
  Saturation/1 -> omegaTC/1, Sum10/2
  Sum10/1 -> Gain1/1
  Gain3/1 -> Sum10/1, Saturation/1  "omegat"
  Integrator/1 -> Gain3/1
  Sum9/1 -> Integrator/1
  tqTurb/1 -> Sum9/2
  tqComp/1 -> Sum9/1
